simulink model "c_lab5_sim"  (R2020b)
settings: Solver=VariableStepAuto  StartTime=0.0  StopTime=100  RelTol=1e-3
libraries: simulink x3
settings Model: Creator=musa oğural  LastModifiedBy=musa oğural

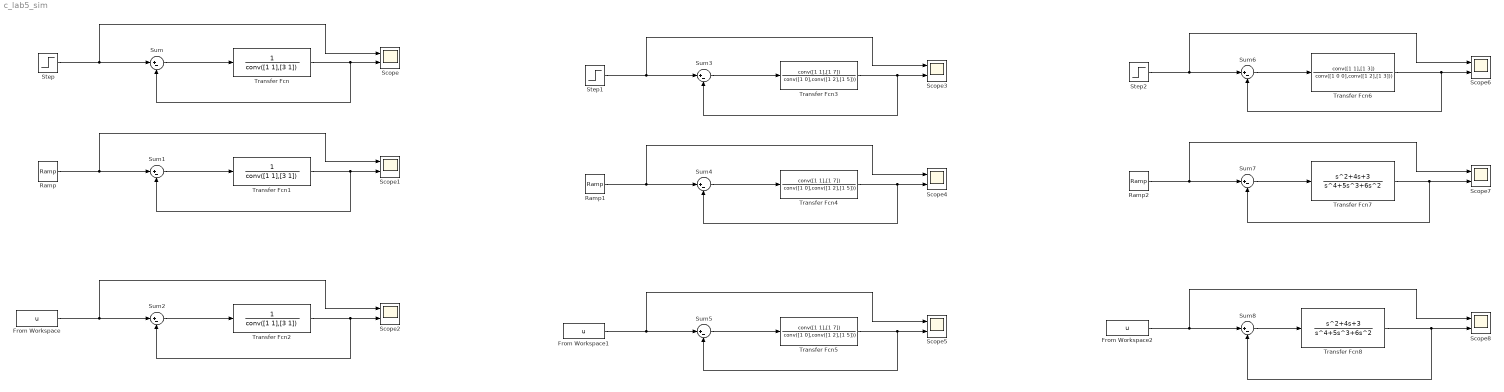
== system c_lab5_sim ==
  From Workspace : FromWorkspace  VariableName=u
  From Workspace1 : FromWorkspace  VariableName=u
  From Workspace2 : FromWorkspace  VariableName=u
  Ramp : simulink/Sources/Ramp  slope=1  start=0  InitialOutput=0
  Ramp1 : simulink/Sources/Ramp  slope=1  start=0  InitialOutput=0
  Ramp2 : simulink/Sources/Ramp  slope=1  start=0  InitialOutput=0
  Scope{,1..8} (9 alike) : Scope  NumInputPorts=2
  Step : Step  Time=0  SampleTime=0
  Step1 : Step  Time=0  SampleTime=0
  Step2 : Step  Time=0  SampleTime=0
  Sum{,1..8} (9 alike) : Sum  Inputs=|+-
  Transfer Fcn : TransferFcn  Denominator=conv([1 1],[3 1])
  Transfer Fcn1 : TransferFcn  Denominator=conv([1 1],[3 1])
  Transfer Fcn2 : TransferFcn  Denominator=conv([1 1],[3 1])
  Transfer Fcn3 : TransferFcn  Numerator=conv([1 1],[1 7])  Denominator=conv([1 0],conv([1 2],[1 5]))
  Transfer Fcn4 : TransferFcn  Numerator=conv([1 1],[1 7])  Denominator=conv([1 0],conv([1 2],[1 5]))
  Transfer Fcn5 : TransferFcn  Numerator=conv([1 1],[1 7])  Denominator=conv([1 0],conv([1 2],[1 5]))
  Transfer Fcn6 : TransferFcn  Numerator=conv([1 1],[1 3])  Denominator=conv([1 0 0],conv([1 2],[1 3]))
  Transfer Fcn7 : TransferFcn  Numerator=[1 4 3 ]  Denominator=[1 5 6 0 0]
  Transfer Fcn8 : TransferFcn  Numerator=[1 4 3 ]  Denominator=[1 5 6 0 0]
  wires:
  Sum/1 -> Transfer Fcn/1
  Step/1 -> Scope/1, Sum/1
  Transfer Fcn/1 -> Sum/2, Scope/2
  Ramp/1 -> Scope1/1, Sum1/1
  Transfer Fcn1/1 -> Sum1/2, Scope1/2
  From Workspace/1 -> Scope2/1, Sum2/1
  Transfer Fcn2/1 -> Sum2/2, Scope2/2
  Sum3/1 -> Transfer Fcn3/1
  From Workspace1/1 -> Scope5/1, Sum5/1
  Ramp1/1 -> Scope4/1, Sum4/1
  Transfer Fcn5/1 -> Sum5/2, Scope5/2
  Transfer Fcn3/1 -> Sum3/2, Scope3/2
  Transfer Fcn4/1 -> Sum4/2, Scope4/2
  Step1/1 -> Scope3/1, Sum3/1
  Sum6/1 -> Transfer Fcn6/1
  From Workspace2/1 -> Scope8/1, Sum8/1
  Ramp2/1 -> Scope7/1, Sum7/1
  Transfer Fcn6/1 -> Sum6/2, Scope6/2
  Step2/1 -> Scope6/1, Sum6/1
  Sum8/1 -> Transfer Fcn8/1
  Transfer Fcn8/1 -> Sum8/2, Scope8/2
  Transfer Fcn7/1 -> Sum7/2, Scope7/2
  Sum7/1 -> Transfer Fcn7/1
  Sum4/1 -> Transfer Fcn4/1
  Sum5/1 -> Transfer Fcn5/1
  Sum1/1 -> Transfer Fcn1/1
  Sum2/1 -> Transfer Fcn2/1
